simulink model "Inverter_Model"  (R2024a)
settings: Solver=ode4  StartTime=0.0  StopTime=25  FixedStep=Ts_power  RelTol=1e-3
undefined symbols (not defined in the file or in its folder): Cdc, ESR_dc, eta_mppt, L_filter, m_ref, n_switches, Rth_ch, Rth_ha, Rth_jc, Rth_jc_hotspot, Tamb, tau_ch, tau_ha, tau_jc, tau_jc_hotspot, Ts_power, Vmppt_max, Vmppt_min
libraries: spsSeriesRLCBranchLib x6, eeRmsMeasurement x2, spspowerguiLib x1, spsPower3phInstantaneousLib x1, spsControlledVoltageSourceLib x1, spsUniversalBridgeLib x1, spsCurrentMeasurementLib x1, spsPWMGenerator2LevelLib x1, spsThreePhaseSeriesRLCLoadLib x1, spsThreePhaseVIMeasurementLib x1, spsVoltageMeasurementLib x1
settings Model: Creator=M Wasib  LastModifiedBy=M Wasib
settings ConfigComp: CovBoundaryAbsTol=1.0e-5

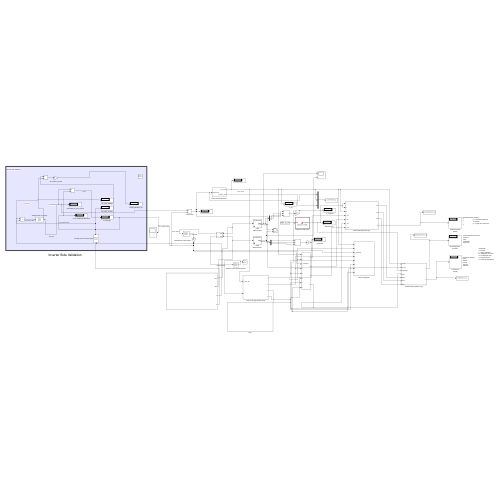
[thumbnail: Simulink's stored preview of the top-level diagram]
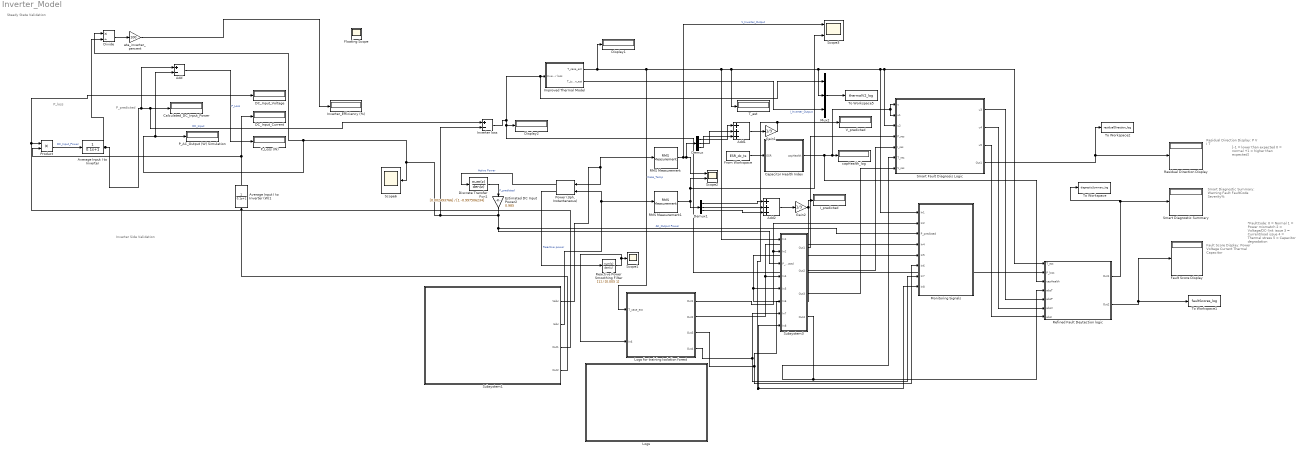
== system Inverter_Model ==
  note: Inverter Side Validation
  note: Steady State Validation
  note: P_predicted
  note: P_loss
  note: [-1 = lower than expected
      |  0 = normal
      | +1 = higher than expected]
  note: Fault Score Display:
      | Power
      | Voltage
      | Current
      | Thermal
      | Capacitor
  note: *FaultCode:
      | 0 = Normal
      | 1 = Power mismatch
      | 2 = Voltage/DC-link issue
      | 3 = Current/load issue
      | 4 = Thermal stress
      | 5 = Capacitor degradation
  note: Residual Direction Display:
      | P
      | V
      | I
      | T
  note: Smart Diagnostic Summary:
      | Warning
      | Fault
      | FaultCode
      | Severity%
  Add : Sum  Inputs=+-
  Add1 : Sum  Inputs=+++
  Add2 : Sum  Inputs=+++
  "Average Input I to Inverter " : TransferFcn  Denominator=[0.1 1]
  Average Input I to Inverter (W)1 : TransferFcn  Denominator=[0.1 1]
  Calculated_DC_Input_Power : Display
  Capacitor Health Index : MATLAB Function  TreatAsAtomicUnit=on
  DC_Input_Current : Display
  DC_Input_Voltage : Display
  Demux : Demux  Outputs=3
  Demux1 : Demux  Outputs=3
  Discrete Transfer Fcn1 : DiscreteTransferFcn  Numerator=[0.002493766]  Denominator=[1 -0.997506234]  InitialStates=9023  RndMeth=Round
  Display1 : Display
  Display2 : Display
  Divide : Product  Inputs=*/
  Estimated DC Input Power2 : Gain  Gain=0.985
  Fault Score Display : Display
  Floating Scope : Scope
      settings: Floating=on
  From Workspace : FromWorkspace  VariableName=ESR_dc_ts
  Gain1 : Gain  Gain=1/3
  Gain2 : Gain  Gain=1/3
  I_predicted : Display
  Improved Thermal Model : Subsystem
  Inverter loss : Sum  Inputs=+-
  Inverter_Efficiency (%) : Display
  Logs : Subsystem
  Logs for training Isolation forest : Subsystem
  Monitoring Signals : Subsystem
  Mux2 : Mux  Inputs=3
  P_AC_Output (W) Simulation : Display
  P_Loss (W) : Display
  "Power (3ph, Instantaneous)" : spsPower3phInstantaneousLib/Power (3ph, Instantaneous)
  Product : Product
  RMS Measurement : eeRmsMeasurement/RMS Measurement  LabelModeActiveChoice=Total  F=60  SpecifyHarmonics=off  K=[0 1 2]  Ts=0
      settings: LibrarySourceBlock=|
      | ee_sl_lib/Measurements/RMS
      | Measurement
  RMS Measurement1 : eeRmsMeasurement/RMS Measurement  LabelModeActiveChoice=Total  F=60  SpecifyHarmonics=off  K=[0 1 2]  Ts=0
      settings: LibrarySourceBlock=|
      | ee_sl_lib/Measurements/RMS
      | Measurement
  Reactive Power Smoothing Filter : TransferFcn  Denominator=[0.005 1]
  Refined Fault Deytection logic : Subsystem
  Residual Direction Display : Display
  Scope1 : Scope
  Scope2 : Scope  NumInputPorts=2
  Scope3 : Scope  NumInputPorts=2
  Scope6 : Scope
  Smart Diagnostic Summary : Display
  Smart Fault Diagnosis Logic : Subsystem
  Subsystem1 : Subsystem
  Subsystem3 : Subsystem
  T_est : Display
  To Workspace : ToWorkspace  VariableName=diagnosticSummary_log  SaveFormat=Timeseries  SampleTime=-1
  To Workspace1 : ToWorkspace  VariableName=faultScores_log  SaveFormat=Timeseries  SampleTime=-1
  To Workspace2 : ToWorkspace  VariableName=residualDirection_log  SaveFormat=Timeseries  SampleTime=-1
  To Workspace5 : ToWorkspace  VariableName=thermalV2_log  SaveFormat=Timeseries  SampleTime=-1
  V_predicted : Display
  capHealth_log : Display
  eta_inverter_percent : Gain  Gain=100
  wires:
  Refined Fault Deytection logic/1(Out1) -> To Workspace/1, Smart Diagnostic Summary/1
  Smart Fault Diagnosis Logic/2(u4) -> Refined Fault Deytection logic/6(absV)
  Smart Fault Diagnosis Logic/3(u5) -> Refined Fault Deytection logic/7(absI)
  Refined Fault Deytection logic/2(Out2) -> To Workspace1/1, Fault Score Display/1
  Gain1/1 -> Subsystem3/8(In8), Monitoring Signals/8(In8), V_predicted/1
  Demux/2 -> Add1/2
  From Workspace/1 -> Capacitor Health Index/1(ESR)
  Gain2/1 -> Subsystem3/5(In5), Monitoring Signals/5(In5), I_predicted/1
  Add1/1 -> Gain1/1
  "Power (3ph, Instantaneous)"/2 -> Reactive Power Smoothing Filter/1  "Reactive power"
  Demux1/1 -> Add2/1
  RMS Measurement1/1 -> Scope2/2, Scope3/2, Demux1/1  "I_Inverter_Output"
  Demux/3 -> Add1/3
  Capacitor Health Index/1(capHealth) -> Smart Fault Diagnosis Logic/2(u1), Smart Fault Diagnosis Logic/1(u), capHealth_log/1, Refined Fault Deytection logic/3(capHealth)
  Logs for training Isolation forest/3(Out3) -> Monitoring Signals/6(In6), Subsystem3/6(In6)
  Logs for training Isolation forest/1(Out1) -> Subsystem3/2(In2), Monitoring Signals/2(In2)
  Logs for training Isolation forest/4(Out4) -> Monitoring Signals/7(In7), Subsystem3/7(In7)
  Logs for training Isolation forest/2(Out2) -> Subsystem3/4(In4), Monitoring Signals/4(In4)
  Demux1/3 -> Add2/3
  "Power (3ph, Instantaneous)"/1 -> Discrete Transfer Fcn1/1  "Active Power"
  Inverter loss/1 -> Mux2/1, Improved Thermal Model/1(Invertor loss), Refined Fault Deytection logic/2(P_loss), Display2/1
  Add2/1 -> Gain2/1
  Reactive Power Smoothing Filter/1 -> Logs for training Isolation forest/2(In6), Scope1/1
  Demux/1 -> Add1/1
  RMS Measurement/1 -> Scope3/1, Scope2/1, Demux/1  "V_Inverter_Output"
  Smart Fault Diagnosis Logic/1(u3) -> Refined Fault Deytection logic/5(absP)
  Demux1/2 -> Add2/2
  Smart Fault Diagnosis Logic/4(Out1) -> To Workspace2/1, Residual Direction Display/1
  Improved Thermal Model/1(T_case_est) -> Display1/1, Subsystem3/1(In1), Smart Fault Diagnosis Logic/3(u2), Refined Fault Deytection logic/1(T_est), Monitoring Signals/1(In1), Mux2/2, T_est/1, Logs for training Isolation forest/1(T_case_est)  "Case_Temp"
  Improved Thermal Model/2(T_junction_est) -> Mux2/3
  Mux2/1 -> To Workspace5/1
  Subsystem1/2(Iabc) -> "Power (3ph, Instantaneous)"/2, RMS Measurement1/1
  Subsystem1/1(Vabc) -> "Power (3ph, Instantaneous)"/1, RMS Measurement/1
  Subsystem3/4(Out4) -> Smart Fault Diagnosis Logic/6(T_res), Refined Fault Deytection logic/4(absT)
  Subsystem3/1(Out1) -> Smart Fault Diagnosis Logic/4(P_res)
  Subsystem3/2(Out2) -> Smart Fault Diagnosis Logic/5(I_res)
  Subsystem3/3(Out3) -> Smart Fault Diagnosis Logic/7(V_res)
  eta_inverter_percent/1 -> Inverter_Efficiency (%)/1
  Divide/1 -> eta_inverter_percent/1
  Subsystem1/3(Out1) -> DC_Input_Voltage/1, Product/1
  Subsystem1/4(Out2) -> Average Input I to Inverter (W)1/1
  Average Input I to Inverter (W)1/1 -> DC_Input_Current/1, Product/2
  Estimated DC Input Power2/1 -> Inverter loss/2, Divide/1, P_AC_Output (W) Simulation/1, Add/2, Scope6/1, Monitoring Signals/3(P_predicted), Subsystem3/3(P_predicted)  "AC_Output Power"
  Discrete Transfer Fcn1/1 -> Estimated DC Input Power2/1  "P_predicted"
  Product/1 -> "Average Input I to Inverter "/1  "DC_Input_Power"
  "Average Input I to Inverter "/1 -> Divide/2, Add/1, Inverter loss/1, Calculated_DC_Input_Power/1  "DC_Input"
  Add/1 -> P_Loss (W)/1  "P_Loss"

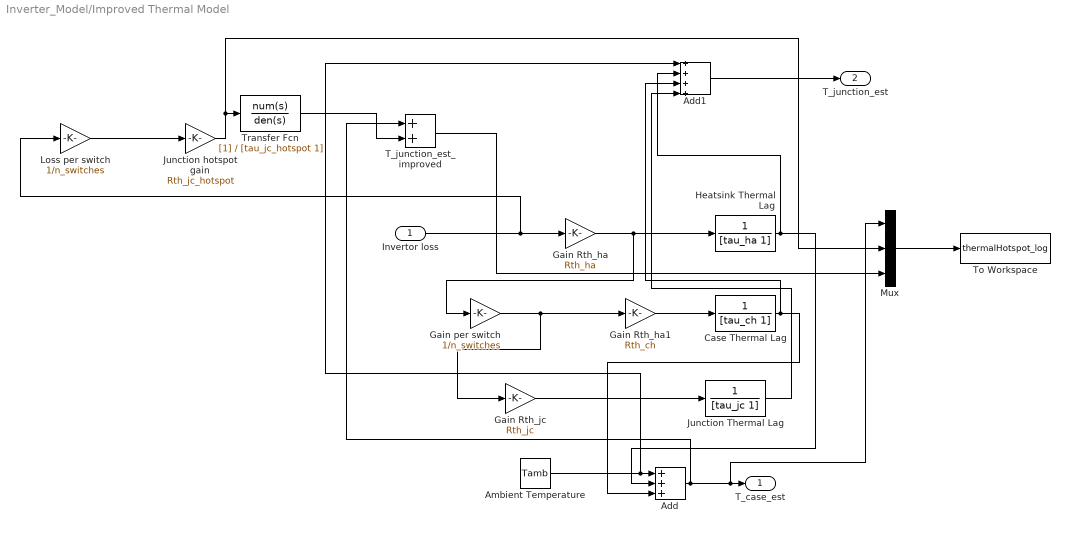
== system Inverter_Model/Improved Thermal Model ==
  Invertor loss : Inport
  Add : Sum  Inputs=+++
  Add1 : Sum  Inputs=++++
  Ambient Temperature : Constant  Value=Tamb
  Case Thermal Lag : TransferFcn  Denominator=[tau_ch 1]
  Gain Rth_ha : Gain  Gain=Rth_ha
  Gain Rth_ha1 : Gain  Gain=Rth_ch
  Gain Rth_jc : Gain  Gain=Rth_jc
  Gain per switch : Gain  Gain=1/n_switches
  Heatsink Thermal Lag : TransferFcn  Denominator=[tau_ha 1]
  Junction Thermal Lag : TransferFcn  Denominator=[tau_jc 1]
  Junction hotspot gain : Gain  Gain=Rth_jc_hotspot
  Loss per switch : Gain  Gain=1/n_switches
  Mux : Mux  Inputs=3
  T_junction_est_improved : Sum
  To Workspace : ToWorkspace  VariableName=thermalHotspot_log  SaveFormat=Timeseries  SampleTime=-1
  Transfer Fcn : TransferFcn  Denominator=[tau_jc_hotspot 1]
  T_case_est : Outport
  T_junction_est : Outport  Port=2
  wires:
  Invertor loss/1 -> Loss per switch/1, Gain Rth_ha/1
  Gain Rth_ha/1 -> Gain per switch/1, Heatsink Thermal Lag/1
  Gain per switch/1 -> Gain Rth_jc/1, Gain Rth_ha1/1
  Gain Rth_ha1/1 -> Case Thermal Lag/1
  Gain Rth_jc/1 -> Junction Thermal Lag/1
  Ambient Temperature/1 -> Add1/1, Add/1
  Heatsink Thermal Lag/1 -> Add1/2, Add/2
  Case Thermal Lag/1 -> Add1/3, Add/3
  Add/1 -> T_junction_est_improved/1, Mux/1, T_case_est/1
  Junction Thermal Lag/1 -> Add1/4
  Loss per switch/1 -> Junction hotspot gain/1
  Junction hotspot gain/1 -> Mux/2, Transfer Fcn/1
  Transfer Fcn/1 -> T_junction_est_improved/2
  Add1/1 -> T_junction_est/1
  Mux/1 -> To Workspace/1
  T_junction_est_improved/1 -> Mux/3

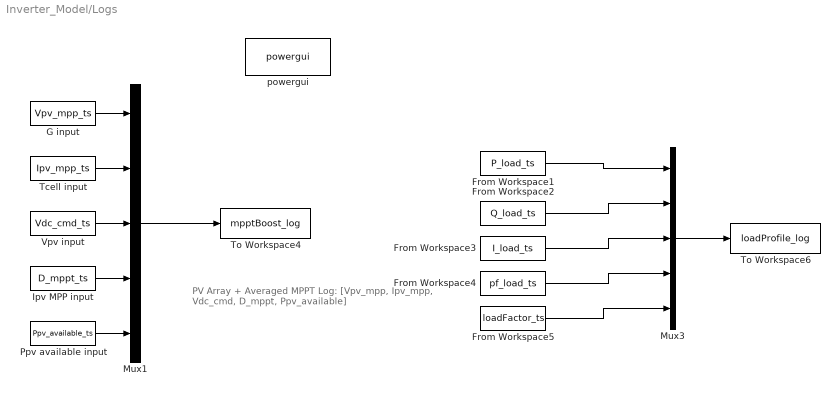
== system Inverter_Model/Logs ==
  note: PV Array + Averaged MPPT Log:
      | [Vpv_mpp, Ipv_mpp, Vdc_cmd, D_mppt, Ppv_available]
  From Workspace1 : FromWorkspace  VariableName=P_load_ts
  From Workspace2 : FromWorkspace  VariableName=Q_load_ts
  From Workspace3 : FromWorkspace  VariableName=I_load_ts
  From Workspace4 : FromWorkspace  VariableName=pf_load_ts
  From Workspace5 : FromWorkspace  VariableName=loadFactor_ts
  G input : FromWorkspace  VariableName=Vpv_mpp_ts
  Ipv MPP input : FromWorkspace  VariableName=D_mppt_ts
  Mux1 : Mux  Inputs=5
  Mux3 : Mux  Inputs=5
  Ppv available input : FromWorkspace  VariableName=Ppv_available_ts
  Tcell input : FromWorkspace  VariableName=Ipv_mpp_ts
  To Workspace4 : ToWorkspace  VariableName=mpptBoost_log  SaveFormat=Timeseries  SampleTime=-1
  To Workspace6 : ToWorkspace  VariableName=loadProfile_log  SaveFormat=Timeseries  SampleTime=-1
  Vpv input : FromWorkspace  VariableName=Vdc_cmd_ts
  powergui : spspowerguiLib/powergui  Priority=1  SimulationMode=Discrete  SampleTime=Ts_power  frequency=60  Iterations=50  frequencyindice=0  Pbase=100e6  ErrMax=1e-4  UnitsV=kV  UnitsW=MW  buscounter=0  FunctionMessages=off  echomessages=off  EnableUseOfTLC=off  CurrentSourceSwitches=off  DisableSnubberDevices=off  DisableRonSwitches=off  DisableVfSwitches=off  DisplayEquations=off  AutomaticDiscreteSolvers=off  SolverType=Tustin/Backward Euler (TBE)  Interpol=off  ExternalGateDelay=off  methode=off  Ts=100  x0status=blocks  SPID=on  SwTol=0  HookPort=off  NonlinearTolerance=1e-4  nMaxIteration=100  ContinueOnMaxIteration=off  RestoreLinks=warning  ResistiveCurrentMeasurement=off  Frange=[0:2:500]  Ylog=off  Xlog=on  ShowGrid=off  save=off  variable=ZData  structure=0  ZoomFFT=off  StartTime=0.0  cycles=1  DisplayStyle=1  fundamental=60  FreqAxis=off  MaxFrequency=1000  frequencyindicesteady=1  RmsSteady=1  display=off
  wires:
  Vpv input/1 -> Mux1/3
  G input/1 -> Mux1/1
  Tcell input/1 -> Mux1/2
  From Workspace5/1 -> Mux3/5
  Ppv available input/1 -> Mux1/5
  From Workspace2/1 -> Mux3/2
  Ipv MPP input/1 -> Mux1/4
  Mux3/1 -> To Workspace6/1
  From Workspace3/1 -> Mux3/3
  Mux1/1 -> To Workspace4/1
  From Workspace1/1 -> Mux3/1
  From Workspace4/1 -> Mux3/4

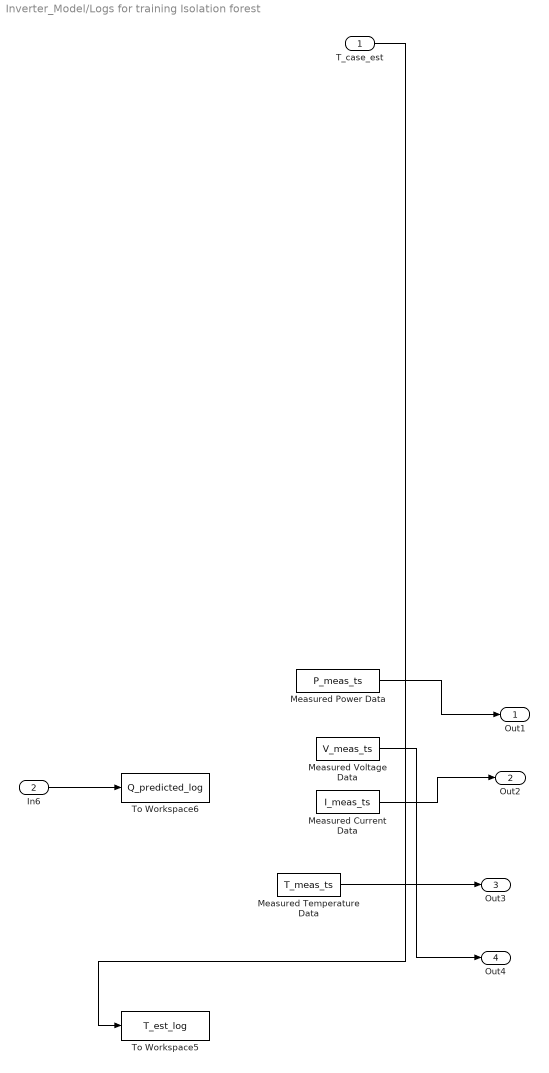
== system Inverter_Model/Logs for training Isolation forest ==
  T_case_est : Inport
  In6 : Inport  Port=2
  Measured Current Data : FromWorkspace  VariableName=I_meas_ts
  Measured Power Data : FromWorkspace  VariableName=P_meas_ts
  Measured Temperature Data : FromWorkspace  VariableName=T_meas_ts
  Measured Voltage Data : FromWorkspace  VariableName=V_meas_ts
  To Workspace5 : ToWorkspace  VariableName=T_est_log  SaveFormat=Timeseries  SampleTime=-1
  To Workspace6 : ToWorkspace  VariableName=Q_predicted_log  SaveFormat=Timeseries  SampleTime=-1
  Out1 : Outport
  Out2 : Outport  Port=2
  Out3 : Outport  Port=3
  Out4 : Outport  Port=4
  wires:
  Measured Temperature Data/1 -> Out3/1
  Measured Voltage Data/1 -> Out4/1
  Measured Current Data/1 -> Out2/1
  Measured Power Data/1 -> Out1/1
  In6/1 -> To Workspace6/1
  T_case_est/1 -> To Workspace5/1

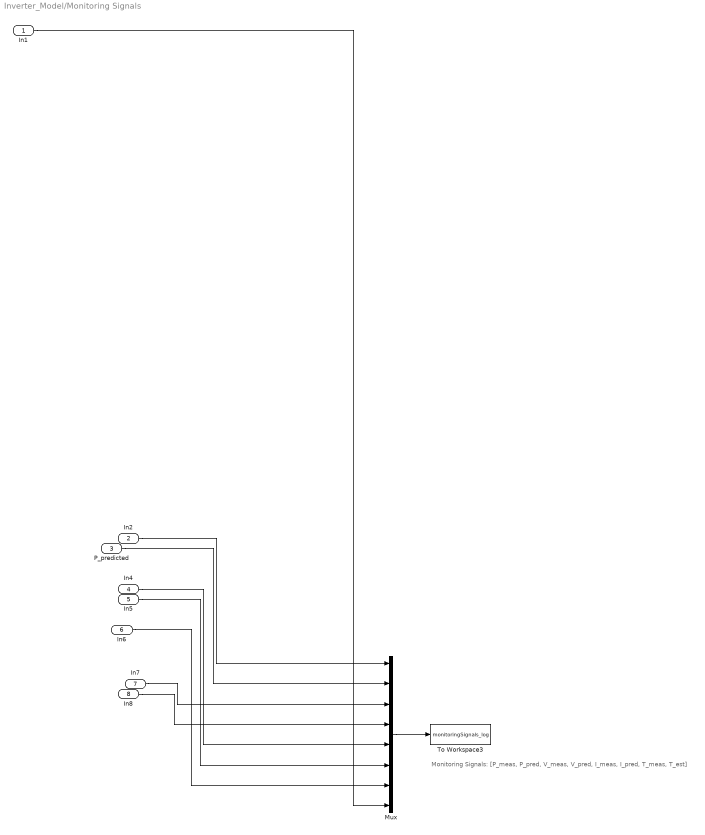
== system Inverter_Model/Monitoring Signals ==
  note: Monitoring Signals:
      | [P_meas, P_pred, V_meas, V_pred, I_meas, I_pred, T_meas, T_est]
  In1 : Inport
  In2 : Inport  Port=2
  P_predicted : Inport  Port=3
  In4 : Inport  Port=4
  In5 : Inport  Port=5
  In6 : Inport  Port=6
  In7 : Inport  Port=7
  In8 : Inport  Port=8
  Mux : Mux  Inputs=8
  To Workspace3 : ToWorkspace  VariableName=monitoringSignals_log  SaveFormat=Timeseries  SampleTime=-1
  wires:
  In1/1 -> Mux/8
  Mux/1 -> To Workspace3/1
  In5/1 -> Mux/6
  In8/1 -> Mux/4
  In6/1 -> Mux/7
  In7/1 -> Mux/3
  In4/1 -> Mux/5
  P_predicted/1 -> Mux/2
  In2/1 -> Mux/1

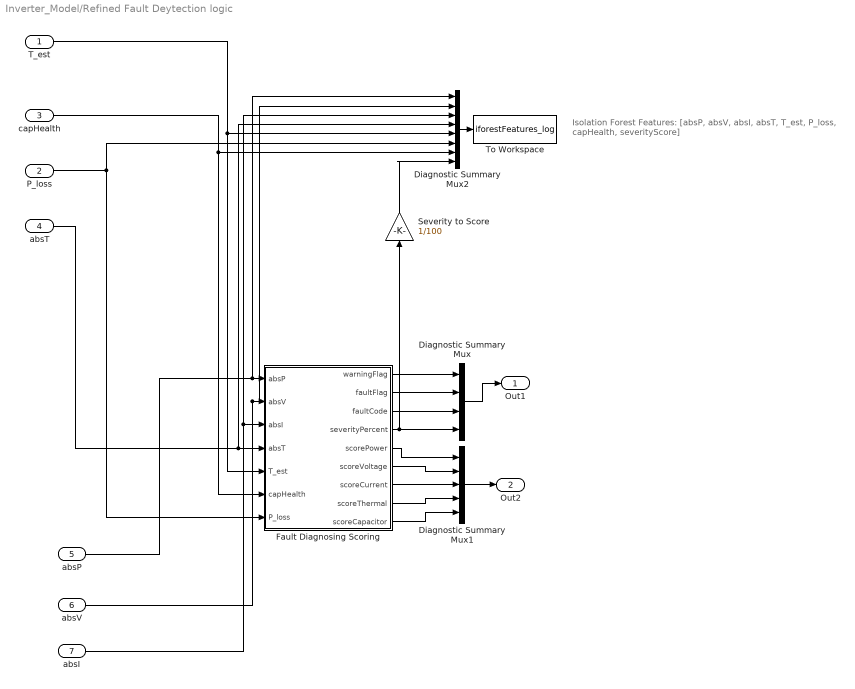
== system Inverter_Model/Refined Fault Deytection logic ==
  note: Isolation Forest Features:
      | [absP, absV, absI, absT, T_est, P_loss, capHealth, severityScore]
  T_est : Inport
  P_loss : Inport  Port=2
  capHealth : Inport  Port=3
  absT : Inport  Port=4
  absP : Inport  Port=5
  absV : Inport  Port=6
  absI : Inport  Port=7
  Diagnostic Summary Mux : Mux
  Diagnostic Summary Mux1 : Mux  Inputs=5
  Diagnostic Summary Mux2 : Mux  Inputs=8
  Fault Diagnosing Scoring : MATLAB Function  TreatAsAtomicUnit=on
  Severity to Score : Gain  Gain=1/100
  To Workspace : ToWorkspace  VariableName=iforestFeatures_log  SaveFormat=Timeseries  SampleTime=-1
  Out1 : Outport
  Out2 : Outport  Port=2
  wires:
  P_loss/1 -> Diagnostic Summary Mux2/6, Fault Diagnosing Scoring/7(P_loss)
  Fault Diagnosing Scoring/6(scoreVoltage) -> Diagnostic Summary Mux1/2
  absV/1 -> Diagnostic Summary Mux2/2, Fault Diagnosing Scoring/2(absV)
  Fault Diagnosing Scoring/4(severityPercent) -> Diagnostic Summary Mux/4, Severity to Score/1
  Fault Diagnosing Scoring/2(faultFlag) -> Diagnostic Summary Mux/2
  Fault Diagnosing Scoring/9(scoreCapacitor) -> Diagnostic Summary Mux1/5
  Fault Diagnosing Scoring/8(scoreThermal) -> Diagnostic Summary Mux1/4
  Fault Diagnosing Scoring/3(faultCode) -> Diagnostic Summary Mux/3
  Fault Diagnosing Scoring/1(warningFlag) -> Diagnostic Summary Mux/1
  Fault Diagnosing Scoring/5(scorePower) -> Diagnostic Summary Mux1/1
  Fault Diagnosing Scoring/7(scoreCurrent) -> Diagnostic Summary Mux1/3
  Diagnostic Summary Mux1/1 -> Out2/1
  capHealth/1 -> Diagnostic Summary Mux2/7, Fault Diagnosing Scoring/6(capHealth)
  absT/1 -> Fault Diagnosing Scoring/4(absT), Diagnostic Summary Mux2/4
  absP/1 -> Diagnostic Summary Mux2/1, Fault Diagnosing Scoring/1(absP)
  T_est/1 -> Diagnostic Summary Mux2/5, Fault Diagnosing Scoring/5(T_est)
  Diagnostic Summary Mux/1 -> Out1/1
  absI/1 -> Diagnostic Summary Mux2/3, Fault Diagnosing Scoring/3(absI)
  Severity to Score/1 -> Diagnostic Summary Mux2/8
  Diagnostic Summary Mux2/1 -> To Workspace/1

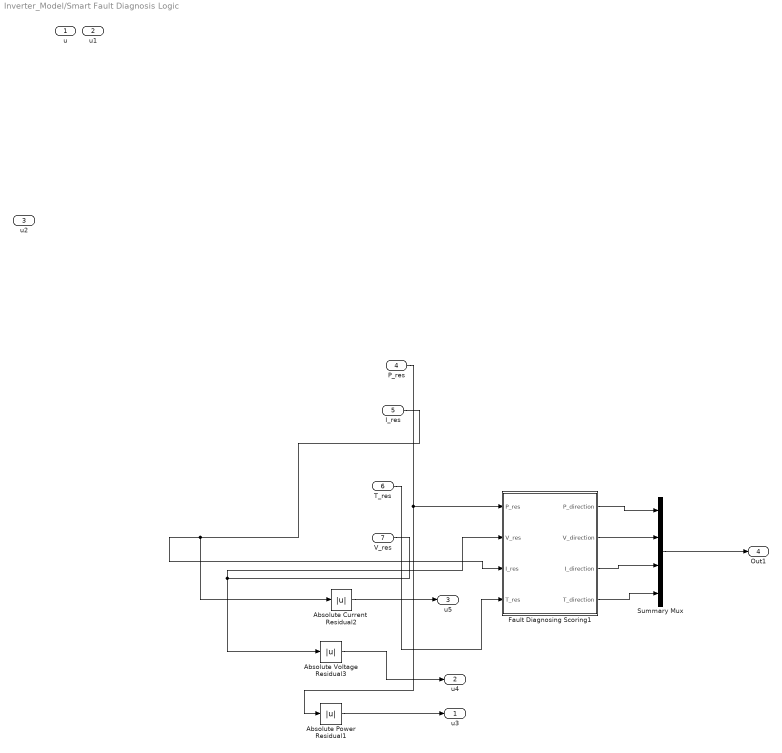
== system Inverter_Model/Smart Fault Diagnosis Logic ==
  u : Inport
  u1 : Inport  Port=2
  u2 : Inport  Port=3
  P_res : Inport  Port=4
  I_res : Inport  Port=5
  T_res : Inport  Port=6
  V_res : Inport  Port=7
  " Summary Mux" : Mux
  Absolute Current  Residual2 : Abs  SaturateOnIntegerOverflow=off
  Absolute Power Residual1 : Abs  SaturateOnIntegerOverflow=off
  Absolute Voltage Residual3 : Abs  SaturateOnIntegerOverflow=off
  Fault Diagnosing Scoring1 : MATLAB Function  TreatAsAtomicUnit=on
  u3 : Outport
  u4 : Outport  Port=2
  u5 : Outport  Port=3
  Out1 : Outport  Port=4
  wires:
  Absolute Voltage Residual3/1 -> u4/1
  Absolute Power Residual1/1 -> u3/1
  T_res/1 -> Fault Diagnosing Scoring1/4(T_res)
  Absolute Current  Residual2/1 -> u5/1
  I_res/1 -> Fault Diagnosing Scoring1/3(I_res), Absolute Current  Residual2/1
  P_res/1 -> Absolute Power Residual1/1, Fault Diagnosing Scoring1/1(P_res)
  V_res/1 -> Absolute Voltage Residual3/1, Fault Diagnosing Scoring1/2(V_res)
  Fault Diagnosing Scoring1/1(P_direction) -> " Summary Mux"/1
  Fault Diagnosing Scoring1/2(V_direction) -> " Summary Mux"/2
  Fault Diagnosing Scoring1/3(I_direction) -> " Summary Mux"/3
  Fault Diagnosing Scoring1/4(T_direction) -> " Summary Mux"/4
  " Summary Mux"/1 -> Out1/1

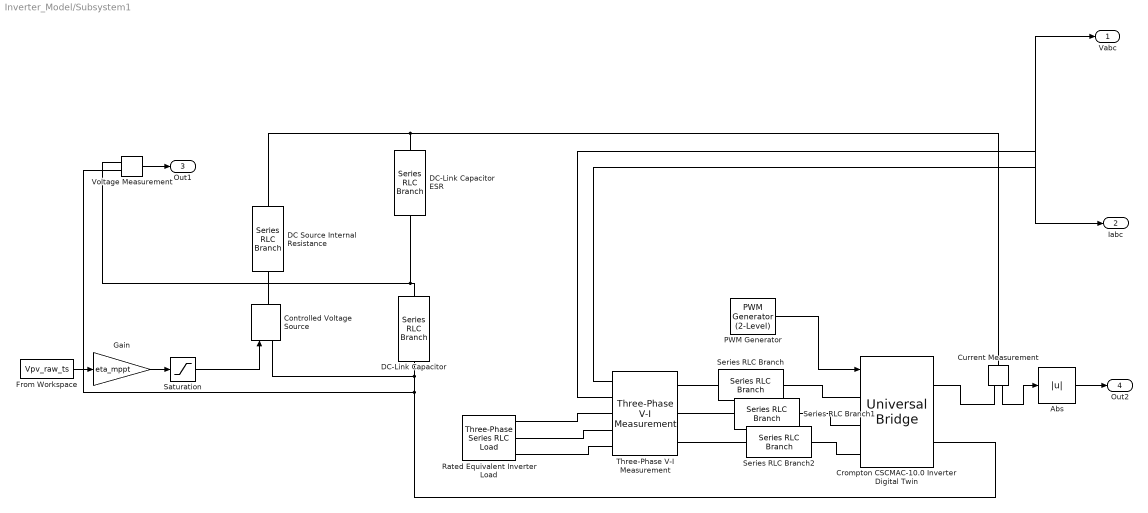
== system Inverter_Model/Subsystem1 ==
  Abs : Abs  SaturateOnIntegerOverflow=off
  Controlled Voltage Source : spsControlledVoltageSourceLib/Controlled Voltage Source  Initialize=on  Source_Type=AC  Amplitude=0  Phase=0  Frequency=0  Measurements=None
  Crompton CSCMAC-10.0 Inverter Digital Twin : spsUniversalBridgeLib/Universal Bridge  Arms=3  SnubberResistance=1e5  SnubberCapacitance=inf  Device=IGBT / Diodes  Ron=1e-3  Lon=0  ForwardVoltages="[  0  0  ]"  ForwardVoltage=0  GTOparameters=[ 10e-6 , 20e-6 ]  IGBTparameters=[ 1e-6 , 2e-6 ]  Measurements=None  Measurements_2=None  converterType=Rectifier
  Current Measurement : spsCurrentMeasurementLib/Current Measurement  PhasorSimulation=off  OutputType=Complex  PSBequivalent=0
  DC Source Internal Resistance : spsSeriesRLCBranchLib/Series RLC Branch  LConnTagsString=__new0  RConnTagsString=__new0  BranchType=R  Resistance=0.01  Inductance=1e-3  SetiL0=off  InitialCurrent=0  Capacitance=1e-6  Setx0=off  InitialVoltage=0  Measurements=None
  DC-Link Capacitor : spsSeriesRLCBranchLib/Series RLC Branch  LConnTagsString=__new0  RConnTagsString=__new0  BranchType=C  Resistance=1  Inductance=1e-3  SetiL0=off  InitialCurrent=0  Capacitance=Cdc  Setx0=off  InitialVoltage=0  Measurements=None
  DC-Link Capacitor ESR : spsSeriesRLCBranchLib/Series RLC Branch  LConnTagsString=__new0  RConnTagsString=__new0  BranchType=R  Resistance=ESR_dc  Inductance=1e-3  SetiL0=off  InitialCurrent=0  Capacitance=1e-6  Setx0=off  InitialVoltage=0  Measurements=None
  From Workspace : FromWorkspace  VariableName=Vpv_raw_ts
  Gain : Gain  Gain=eta_mppt
  "PWM Generator " : spsPWMGenerator2LevelLib/PWM Generator (2-Level)  ModulatorType=Three-phase bridge (6 pulses)  ModulatorMode=Unsynchronized  Fc=fsw  Pc=90  nF=27  MinMax="[ -1  1 ]"  SamplingTechnique=Natural  ModulatingSignals=on  m=m_ref  Freq=fout_ref  Phase=0  Ts=Ts_power  ShowCarrierOutport=off
  Rated Equivalent Inverter Load : spsThreePhaseSeriesRLCLoadLib/Three-Phase Series RLC Load  LConnTagsString=A|B|C  Configuration=Y (grounded)  NominalVoltage=Vll_rated  Vabc=[1e3 1e3 1e3]  Vabcp=[1e3 1e3 1e3]  NominalFrequency=fout_ref  UnbalancedPower=off  ActivePower=P_load_for_sim  InductivePower=Q_load_for_sim  CapacitivePower=0  Pabc=[10e3 9e3 11e3]  QLabc=[100 90 110]  QCabc=[100 90 110]  Pabcp=[10e3 9e3 11e3]  QLabcp=[100 90 110]  QCabcp=[100 90 110]  Measurements=None  LoadType=constant Z
  Saturation : Saturate  UpperLimit=Vmppt_max  LowerLimit=Vmppt_min
  Series RLC Branch : spsSeriesRLCBranchLib/Series RLC Branch  LConnTagsString=__new0  RConnTagsString=__new0  BranchType=RL  Resistance=0.01  Inductance=L_filter  SetiL0=off  InitialCurrent=0  Capacitance=1e-6  Setx0=off  InitialVoltage=0  Measurements=None
  Series RLC Branch1 : spsSeriesRLCBranchLib/Series RLC Branch  LConnTagsString=__new0  RConnTagsString=__new0  BranchType=RL  Resistance=0.01  Inductance=L_filter  SetiL0=off  InitialCurrent=0  Capacitance=1e-6  Setx0=off  InitialVoltage=0  Measurements=None
  Series RLC Branch2 : spsSeriesRLCBranchLib/Series RLC Branch  LConnTagsString=__new0  RConnTagsString=__new0  BranchType=RL  Resistance=0.01  Inductance=L_filter  SetiL0=off  InitialCurrent=0  Capacitance=1e-6  Setx0=off  InitialVoltage=0  Measurements=None
  Three-Phase V-I Measurement : spsThreePhaseVIMeasurementLib/Three-Phase V-I Measurement  VoltageMeasurement=phase-to-ground  SetLabelV=off  LabelV=Vabc  Vpu=off  VpuLL=off  CurrentMeasurement=yes  SetLabelI=off  LabelI=Iabc  Ipu=off  Pbase=100e6  Vbase=500e3  OutputType=Complex  PhasorSimulation=off  PSBequivalent=0
  Voltage Measurement : spsVoltageMeasurementLib/Voltage Measurement  PhasorSimulation=off  OutputType=Complex  PSBequivalent=0
  Vabc : Outport
  Iabc : Outport  Port=2
  Out1 : Outport  Port=3
  Out2 : Outport  Port=4
  wires:
  "PWM Generator "/1 -> Crompton CSCMAC-10.0 Inverter Digital Twin/1
  Saturation/1 -> Controlled Voltage Source/1
  From Workspace/1 -> Gain/1
  Three-Phase V-I Measurement/1 -> Vabc/1
  Three-Phase V-I Measurement/2 -> Iabc/1
  Gain/1 -> Saturation/1
  Voltage Measurement/1 -> Out1/1
  Current Measurement/1 -> Abs/1
  Abs/1 -> Out2/1
  connections:
  Series RLC Branch2/RConn1 -- Crompton CSCMAC-10.0 Inverter Digital Twin/LConn3
  Crompton CSCMAC-10.0 Inverter Digital Twin/RConn2 -- DC-Link Capacitor/RConn1 -- Controlled Voltage Source/LConn1 -- Voltage Measurement/LConn2
  DC Source Internal Resistance/RConn1 -- Current Measurement/LConn1 -- DC-Link Capacitor ESR/RConn1
  Series RLC Branch/LConn1 -- Three-Phase V-I Measurement/LConn1
  Series RLC Branch1/RConn1 -- Crompton CSCMAC-10.0 Inverter Digital Twin/LConn2
  Series RLC Branch1/LConn1 -- Three-Phase V-I Measurement/LConn2
  Series RLC Branch2/LConn1 -- Three-Phase V-I Measurement/LConn3
  Three-Phase V-I Measurement/RConn2 -- Rated Equivalent Inverter Load/LConn2
  Series RLC Branch/RConn1 -- Crompton CSCMAC-10.0 Inverter Digital Twin/LConn1
  Controlled Voltage Source/RConn1 -- DC Source Internal Resistance/LConn1
  Three-Phase V-I Measurement/RConn1 -- Rated Equivalent Inverter Load/LConn1
  Rated Equivalent Inverter Load/LConn3 -- Three-Phase V-I Measurement/RConn3
  Voltage Measurement/LConn1 -- DC-Link Capacitor ESR/LConn1 -- DC-Link Capacitor/LConn1
  Crompton CSCMAC-10.0 Inverter Digital Twin/RConn1 -- Current Measurement/RConn1

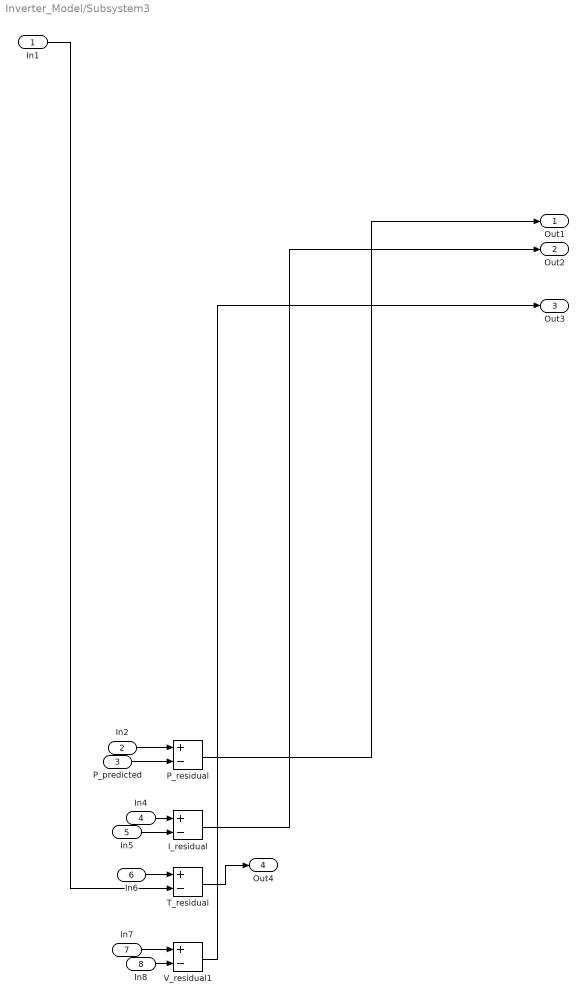
== system Inverter_Model/Subsystem3 ==
  In1 : Inport
  In2 : Inport  Port=2
  P_predicted : Inport  Port=3
  In4 : Inport  Port=4
  In5 : Inport  Port=5
  In6 : Inport  Port=6
  In7 : Inport  Port=7
  In8 : Inport  Port=8
  I_residual : Sum  Inputs=+-
  P_residual : Sum  Inputs=+-
  T_residual : Sum  Inputs=+-
  V_residual1 : Sum  Inputs=+-
  Out1 : Outport
  Out2 : Outport  Port=2
  Out3 : Outport  Port=3
  Out4 : Outport  Port=4
  wires:
  In1/1 -> T_residual/2
  In7/1 -> V_residual1/1
  T_residual/1 -> Out4/1
  In5/1 -> I_residual/2
  In2/1 -> P_residual/1
  V_residual1/1 -> Out3/1
  P_residual/1 -> Out1/1
  I_residual/1 -> Out2/1
  In6/1 -> T_residual/1
  P_predicted/1 -> P_residual/2
  In8/1 -> V_residual1/2
  In4/1 -> I_residual/1

== matlab function Inverter_Model/Smart Fault Diagnosis Logic/Fault Diagnosing Scoring1 ==
  data: P_res input; P_direction output; V_res input; I_res input; T_res input; V_direction output; I_direction output; T_direction output
function [P_direction, V_direction, I_direction, T_direction] = residual_direction(P_res, V_res, I_res, T_res)

% Direction codes:
% -1 = lower than expected
%  0 = normal
% +1 = higher than expected

P_tol = 500;   % W
V_tol = 20;    % V
I_tol = 2;     % A
T_tol = 8;     % degC

P_direction = 0;
V_direction = 0;
I_direction = 0;
T_direction = 0;

if P_res > P_tol
    P_direction = 1;
elseif P_res < -P_tol
    P_direction = -1;
end

if V_res > V_tol
    V_direction = 1;
elseif V_res < -V_tol
    V_direction = -1;
end

if I_res > I_tol
    I_direction = 1;
elseif I_res < -I_tol
    I_direction = -1;
end

if T_res > T_tol
    T_direction = 1;
elseif T_res < -T_tol
    T_direction = -1;
end

end

== matlab function Inverter_Model/Capacitor Health Index ==
  data: ESR input; capHealth output
function capHealth = capacitor_health(ESR)
ESR0 = 0.05;
ESRfault = 0.20;

capHealth = 1 - (ESR - ESR0)/(ESRfault - ESR0);

if capHealth > 1
    capHealth = 1;
end

if capHealth < 0
    capHealth = 0;
end
end

== matlab function Inverter_Model/Refined Fault Deytection logic/Fault Diagnosing Scoring ==
  data: absP input; warningFlag output; absV input; absI input; absT input; T_est input; capHealth input; P_loss input; faultFlag output; faultCode output; severityPercent output; scorePower output; scoreVoltage output; scoreCurrent output; scoreThermal output; scoreCapacitor output
function [warningFlag, faultFlag, faultCode, severityPercent, ...
          scorePower, scoreVoltage, scoreCurrent, scoreThermal, scoreCapacitor] = ...
          fault_diagnosis_score(absP, absV, absI, absT, T_est, capHealth, P_loss)

% Fault codes:
% 0 = Normal
% 1 = Power mismatch
% 2 = Voltage / DC-link issue
% 3 = Current / load issue
% 4 = Thermal stress
% 5 = Capacitor degradation

% Thresholds
P_res_fault = 1000;      % W
V_res_fault = 40;        % V
I_res_fault = 4;         % A
T_res_fault = 15;        % degC
T_warn = 70;             % degC
T_fault = 85;            % degC

% Decision thresholds
warningThreshold = 0.5;
faultThreshold = 1.0;

% Normalize residuals
pN = absP / P_res_fault;
vN = absV / V_res_fault;
iN = absI / I_res_fault;
tN = absT / T_res_fault;

% Temperature score based on estimated inverter temperature
if T_est <= T_warn
    tempN = 0;
else
    tempN = (T_est - T_warn) / (T_fault - T_warn);
end

% Capacitor degradation score
capDeg = 1 - capHealth;

% Keep cap degradation inside valid range
capDeg = min(max(capDeg, 0), 1);

% Fault signature scores
scorePower = pN;
scoreVoltage = 0.6*vN + 0.4*pN;
scoreCurrent = 0.7*iN + 0.3*pN;
scoreThermal = 0.6*tempN + 0.4*tN;
scoreCapacitor = 1.2*capDeg + 0.25*vN + 0.15*pN;

% Limit scores between 0 and 2
scorePower = min(max(scorePower, 0), 2);
scoreVoltage = min(max(scoreVoltage, 0), 2);
scoreCurrent = min(max(scoreCurrent, 0), 2);
scoreThermal = min(max(scoreThermal, 0), 2);
scoreCapacitor = min(max(scoreCapacitor, 0), 2);

% Find strongest fault pattern
scores = [scorePower, scoreVoltage, scoreCurrent, scoreThermal, scoreCapacitor];
[maxScore, maxIndex] = max(scores);

% Raw severity before deadband
rawSeverity = min((maxScore / 2) * 100, 100);

% Default outputs
warningFlag = 0;
faultFlag = 0;
faultCode = 0;
severityPercent = 0;

% Decision logic with healthy deadband
if maxScore < warningThreshold

    % Healthy region: small residuals are ignored
    warningFlag = 0;
    faultFlag = 0;
    faultCode = 0;
    severityPercent = 0;

else

    % Warning or fault region
    warningFlag = 1;
    severityPercent = rawSeverity;

    % Fault code follows strongest score
    faultCode = maxIndex;

    if maxScore >= faultThreshold
        faultFlag = 1;
    else
        faultFlag = 0;
    end

end

% Keep P_loss input active for Simulink/code generation compatibility
unusedLoss = P_loss; %#ok<NASGU>

end
